simulink model "Testailu_1stOrderDelay_vainSimu"  (R2016b)
settings: Solver=ode4  StartTime=0.0  StopTime=max(timeVector)  FixedStep=0.5  RelTol=1e-3
values from neighbouring files (symbols this model uses):
  t_delay_init = 1500    [dsa.m]
  Tau = 3700    [dsa.m]
  TotRange = abs(Values2 - Values1)    [dsa.m]
settings Model: Creator=maki9  LastModifiedBy=maki9

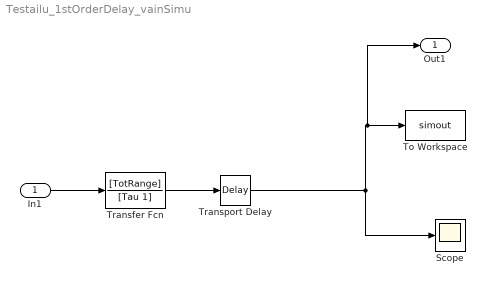
== system Testailu_1stOrderDelay_vainSimu ==
  In1 : Inport
  Scope : Scope
  To Workspace : ToWorkspace  VariableName=simout  SaveFormat=Timeseries  SampleTime=-1
  Transfer Fcn : TransferFcn  Numerator=[TotRange]  Denominator=[Tau 1]
  Transport Delay : TransportDelay  DelayTime=t_delay_init
  Out1 : Outport
  wires:
  Transport Delay/1 -> Out1/1, To Workspace/1, Scope/1
  In1/1 -> Transfer Fcn/1
  Transfer Fcn/1 -> Transport Delay/1
